simulink model "ellipse_animation"  (Simulink 8.3)
settings: Solver=ode45  StartTime=0.0  StopTime=10000  RelTol=1e-3
undefined symbols (not defined in the file or in its folder): drawEllipse
libraries: simulink x1
settings Model: Creator=beard  LastModifiedBy=jhl48
settings OptimizationCC: ExpressionDepthLimit=2147483647  InitFltsAndDblsToZero=on
settings DebuggingCC: FcnCallInpInsideContextMsg=UseLocalSettings

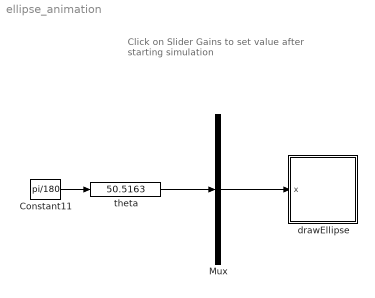
== system ellipse_animation ==
  note: Click on Slider Gains to set value
      | after starting simulation
  Constant11 : Constant  Value=pi/180
  Mux : Mux  Inputs=1
  drawEllipse : Subsystem
      mask init:
      | % drawing parameters
      | L = 1;
      | gap = 0.01;
      | width = 1.0;
      | height = 0.1;
      mask Display: image(imread('tv.jpg'))
  theta : simulink/Math Operations/Slider Gain  low=-180  gain=50.5163  high=180
  wires:
  Constant11/1 -> theta/1
  Mux/1 -> drawEllipse/1(x)
  theta/1 -> Mux/1

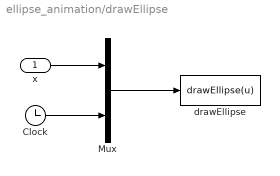
== system ellipse_animation/drawEllipse ==
  x : Inport
  Clock : Clock
  Mux : Mux  Inputs=2
  drawEllipse : MATLABFcn  MATLABFcn=drawEllipse(u)  OutputDimensions=0  SampleTime=0.1
  wires:
  Mux/1 -> drawEllipse/1
  x/1 -> Mux/1
  Clock/1 -> Mux/2
